simulink model "MCU_State"  (R2022b)
settings: Solver=FixedStepDiscrete  StartTime=0.0  StopTime=10.0  FixedStep=0.002  RelTol=1e-3
undefined symbols (not defined in the file or in its folder): cNoneMode, cSingleBoardMode, FAULT, POWER_ON, STANDBY, WORKING
settings Model: DataDictionary=MCU_Stateflow_Datadictionary_objects.sldd  Creator=ZYH  LastModifiedBy=ZYH
settings OptimizationCC: DefaultParameterBehavior=Inlined  EnhancedBackFolding=on  PassReuseOutputArgsAs=Individual arguments  ZeroExternalMemoryAtStartup=off  ZeroInternalMemoryAtStartup=off  OptimizeBlockOrder=speed  DifferentSizesBufferReuse=on  OptimizationCustomize=off  EfficientTunableParamExpr=on
settings DebuggingCC: ParameterTunabilityLossMsg=error
settings SFSimCC: MATLABDynamicMemAlloc=off
settings RTWCC: Description=Embedded Coder  SystemTargetFile=ert.tlc  GenCodeOnly=on  TemplateMakefile=ert_default_tmf
settings CodeAppCC: ForceParamTrailComments=on  IgnoreCustomStorageClasses=off  OperatorAnnotations=on  SimulinkDataObjDesc=on  SFDataObjDesc=on  InsertBlockDesc=on
settings ERTTargetCC: TargetLangStandard=C99 (ISO)  GenerateSampleERTMain=on  InlinedParameterPlacement=NonHierarchical  ERTCustomFileTemplate=example_file_process.tlc

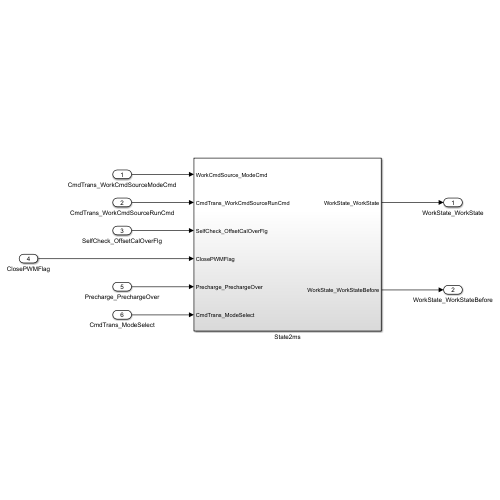
[thumbnail: Simulink's stored preview of the top-level diagram]
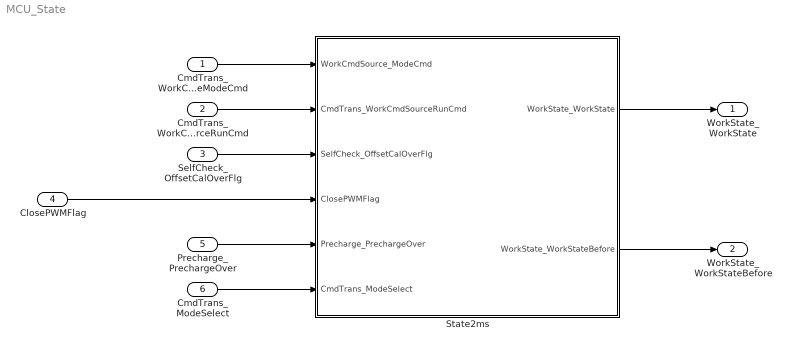
== system MCU_State ==
  CmdTrans_WorkCmdSourceModeCmd : Inport
  CmdTrans_WorkCmdSourceRunCmd : Inport  Port=2
  SelfCheck_OffsetCalOverFlg : Inport  Port=3
  ClosePWMFlag : Inport  Port=4
  Precharge_PrechargeOver : Inport  Port=5
  CmdTrans_ModeSelect : Inport  Port=6
  State2ms : Subsystem
      settings: RTWSystemCode=Nonreusable function
  WorkState_WorkState : Outport
  WorkState_WorkStateBefore : Outport  Port=2
  wires:
  SelfCheck_OffsetCalOverFlg/1 -> State2ms/3(SelfCheck_OffsetCalOverFlg)
  Precharge_PrechargeOver/1 -> State2ms/5(Precharge_PrechargeOver)
  CmdTrans_WorkCmdSourceRunCmd/1 -> State2ms/2(CmdTrans_WorkCmdSourceRunCmd)
  State2ms/1(WorkState_WorkState) -> WorkState_WorkState/1
  State2ms/2(WorkState_WorkStateBefore) -> WorkState_WorkStateBefore/1
  CmdTrans_WorkCmdSourceModeCmd/1 -> State2ms/1(WorkCmdSource_ModeCmd)
  CmdTrans_ModeSelect/1 -> State2ms/6(CmdTrans_ModeSelect)
  ClosePWMFlag/1 -> State2ms/4(ClosePWMFlag)

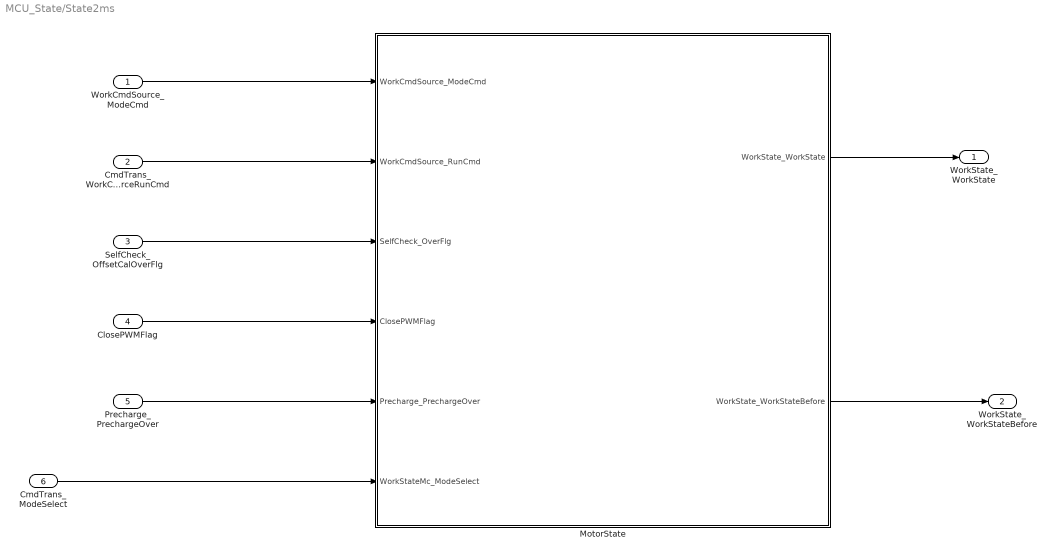
== system MCU_State/State2ms ==
  WorkCmdSource_ModeCmd : Inport
  CmdTrans_WorkCmdSourceRunCmd : Inport  Port=2
  SelfCheck_OffsetCalOverFlg : Inport  Port=3
  ClosePWMFlag : Inport  Port=4
  Precharge_PrechargeOver : Inport  Port=5
  CmdTrans_ModeSelect : Inport  Port=6
  MotorState : Stateflow chart  TreatAsAtomicUnit=on
      settings: RTWSystemCode=Reusable function  PortSchema="{\"entries\":[{\"content\":{\"sides\":[{\"content\":{\"connectorIds\":[\"In4\",\"In3\",\"In1\",\"In2\",\"In5\",\"In6\"]},\"type\":\"ConnectorPlacement.EquallySpacedRectSide\",\"uuid\":\"e0adab7d-9c82-44fd-b38c-331bb9d71454\"},{\"content\":{\"connectorIds\":[\"Out1\",\"Out2\"],\"side\":\"RIGHT\"},\"type\":\"ConnectorPlacement.EquallySpacedRectSide\",\"uuid\":\"98ad1acc-debf-46f0-91aa-4bd2062f60b6\"},{\"content\":{\"connectorIds\":[],\"side\":\"TOP\"},\"type\":\"ConnectorPlacement.EquallySpacedRectSide\",\"uuid\":\"a7c2d312-245c-4ce1-bea5-1bac95c515f1\"},{\"content\":{\"connectorIds\":[],\"side\":\"BOTTOM\"},\"type\":\"ConnectorPlacement.EquallySpacedRectSide\",\"uuid\":\"175f3b6b-1019-4e6e-83d9-bf4c82f74bc8\"}]},\"type\":\"ConnectorPlacement.EquallySpacedConnector\",\"uuid\":\"df312d8c-c57e-4b1a-958b-330641c1b4d1\"}],\"packageUris\":[\"http://schema.mathworks.com/mf0/Connector/R2020b\"],\"version\":\"1.0\"}"
  WorkState_WorkState : Outport
  WorkState_WorkStateBefore : Outport  Port=2
  wires:
  SelfCheck_OffsetCalOverFlg/1 -> MotorState/1(SelfCheck_OverFlg)
  Precharge_PrechargeOver/1 -> MotorState/5(Precharge_PrechargeOver)
  CmdTrans_WorkCmdSourceRunCmd/1 -> MotorState/3(WorkCmdSource_RunCmd)
  MotorState/1(WorkState_WorkState) -> WorkState_WorkState/1
  MotorState/2(WorkState_WorkStateBefore) -> WorkState_WorkStateBefore/1
  WorkCmdSource_ModeCmd/1 -> MotorState/4(WorkCmdSource_ModeCmd)
  CmdTrans_ModeSelect/1 -> MotorState/6(WorkStateMc_ModeSelect)
  ClosePWMFlag/1 -> MotorState/2(ClosePWMFlag)

== stateflow chart MCU_State/State2ms/MotorState ==
  state PowerOn
    %包含零漂校正和ctrl_reset
    WorkState_WorkState = POWER_ON;
  state Fault
  state StandBy
    WorkState_WorkState = STANDBY;
  state Working
    WorkState_WorkState = WORKING;
  (default) -> PowerOn
  PowerOn -> (junction 21) : [SelfCheck_OverFlg == 1]
  (junction 13) -> Fault : {
      | WorkState_WorkState = FAULT;
      | WorkState_WorkStateBefore = POWER_ON;
      | %WorkState_ModeSelect = cNoneMode;
      | }
  (junction 21) -> (junction 13) [order 1] : [ClosePWMFlag == 1]
  (junction 21) -> StandBy [order 2] : {
      | WorkState_WorkState = STANDBY;
      | WorkState_WorkStateBefore = POWER_ON;
      | %WorkState_ModeSelect = cNoneMode;
      | }
  StandBy -> (junction 26) [order 1] : [ClosePWMFlag ==1]
  (junction 26) -> Fault : {
      | WorkState_WorkState = FAULT;
      | WorkState_WorkStateBefore = STANDBY;
      | %WorkState_ModeSelect = cNoneMode
      | }
  Fault -> (junction 47) : [ClosePWMFlag ==0]
  (junction 47) -> StandBy : {
      | WorkState_WorkState = STANDBY;
      | WorkState_WorkStateBefore = FAULT;
      | %WorkState_ModeSelect = cNoneMode
      | }
  StandBy -> (junction 30) [order 2] : [(WorkCmdSource_ModeCmd ~=cNoneMode & WorkCmdSource_RunCmd==true &Precharge_PrechargeOver==true) ||(WorkCmdSource_ModeCmd ==cSingleBoardMode)]
  (junction 72) -> StandBy : {
      | WorkState_WorkState = STANDBY;
      | WorkState_WorkStateBefore = POWER_ON;
      | %WorkState_ModeSelect = cNoneMode;
      | }
  (junction 30) -> Working : {WorkState_WorkState =WORKING;
      | WorkState_WorkStateBefore = STANDBY;}
  Working -> (junction 72) [order 2] : %[(WorkCmdSource_RunCmd ==false & WorkState_ModeSelect ~= cSingleBoardMode) || (WorkState_ModeSelect == cNoneMode)]
      | [(WorkCmdSource_RunCmd ==false & WorkStateMc_ModeSelect ~= cSingleBoardMode) || (WorkStateMc_ModeSelect == cNoneMode)]
  (junction 43) -> Fault : {WorkState_WorkState = FAULT;
      | WorkState_WorkStateBefore = WORKING;
      | %WorkState_ModeSelect = cNoneMode;
      | }
  Working -> (junction 43) [order 1] : [ClosePWMFlag==1]
  data: SelfCheck_OverFlg input; POWER_ON parameter; ClosePWMFlag input; FAULT parameter; WorkState_WorkState output; WorkState_WorkStateBefore output; cNoneMode parameter; STANDBY parameter; cSingleBoardMode parameter; WorkCmdSource_RunCmd input; WorkCmdSource_ModeCmd input; Precharge_PrechargeOver input; WORKING parameter; WorkStateMc_ModeSelect input
